simulink model "Environment"  (R2012b)
settings: Solver=FixedStepDiscrete  StartTime=0.0  StopTime=500  FixedStep=0.1  RelTol=1e-3
values from neighbouring files (symbols this model uses):
  tank1_cross_section_area_m2 = 1    [constants.m]
  tank1_max_vol_m3 = 7    [constants.m]
  tank1_pump_flow_rate_m3s = 0.2    [constants.m]
  tank1_sensor_hi_height_m = 5    [constants.m]
  tank1_sensor_lo_height_m = 2    [constants.m]
  tank1_valve_flow_rate_m3s = 0.1    [constants.m]
  tank2_cross_section_area_m2 = 2    [constants.m]
  tank2_e_valve_flow_rate_m3s = 0.2    [constants.m]
  tank2_max_vol_m3 = 8    [constants.m]
  tank2_p_valve_flow_rate_m3s = 0.05    [constants.m]
  tank2_sensor_hi_height_m = 3    [constants.m]
  tank2_sensor_lo_height_m = 1    [constants.m]
  tank2_sensor_md_height_m = 2    [constants.m]
  time_increment_s = 0.1    [constants.m]
settings Model: Creator=Kerianne  LastModifiedBy=Kerianne
settings DataIOCC: SaveFormat=Structure
settings OptimizationCC: InlineParams=on

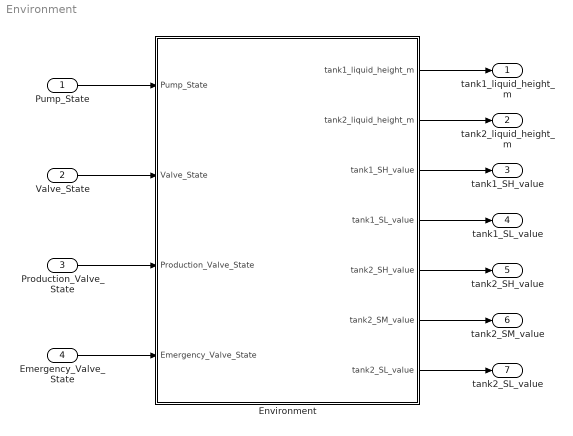
== system Environment ==
  Pump_State : Inport
  Valve_State : Inport  Port=2
  Production_Valve_State : Inport  Port=3
  Emergency_Valve_State : Inport  Port=4
  Environment : Subsystem
  tank1_liquid_height_m : Outport
  tank2_liquid_height_m : Outport  Port=2
  tank1_SH_value : Outport  Port=3
  tank1_SL_value : Outport  Port=4
  tank2_SH_value : Outport  Port=5
  tank2_SM_value : Outport  Port=6
  tank2_SL_value : Outport  Port=7
  wires:
  Pump_State/1 -> Environment/1(Pump_State)
  Valve_State/1 -> Environment/2(Valve_State)
  Production_Valve_State/1 -> Environment/3(Production_Valve_State)
  Emergency_Valve_State/1 -> Environment/4(Emergency_Valve_State)
  Environment/1(tank1_liquid_height_m) -> tank1_liquid_height_m/1
  Environment/2(tank2_liquid_height_m) -> tank2_liquid_height_m/1
  Environment/3(tank1_SH_value) -> tank1_SH_value/1
  Environment/4(tank1_SL_value) -> tank1_SL_value/1
  Environment/5(tank2_SH_value) -> tank2_SH_value/1
  Environment/6(tank2_SM_value) -> tank2_SM_value/1
  Environment/7(tank2_SL_value) -> tank2_SL_value/1

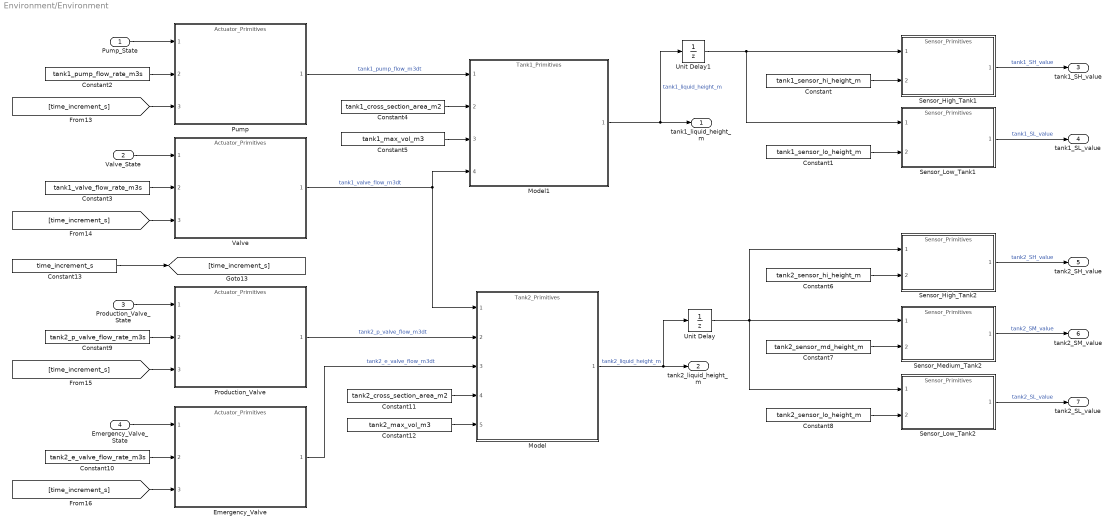
== system Environment/Environment ==
  Pump_State : Inport
  Valve_State : Inport  Port=2
  Production_Valve_State : Inport  Port=3
  Emergency_Valve_State : Inport  Port=4
  Constant : Constant  Value=tank1_sensor_hi_height_m
  Constant1 : Constant  Value=tank1_sensor_lo_height_m
  Constant10 : Constant  Value=tank2_e_valve_flow_rate_m3s
  Constant11 : Constant  Value=tank2_cross_section_area_m2
  Constant12 : Constant  Value=tank2_max_vol_m3
  Constant13 : Constant  Value=time_increment_s
  Constant2 : Constant  Value=tank1_pump_flow_rate_m3s
  Constant3 : Constant  Value=tank1_valve_flow_rate_m3s
  Constant4 : Constant  Value=tank1_cross_section_area_m2
  Constant5 : Constant  Value=tank1_max_vol_m3
  Constant6 : Constant  Value=tank2_sensor_hi_height_m
  Constant7 : Constant  Value=tank2_sensor_md_height_m
  Constant8 : Constant  Value=tank2_sensor_lo_height_m
  Constant9 : Constant  Value=tank2_p_valve_flow_rate_m3s
  Emergency_Valve : ModelReference  ModelNameDialog=Actuator_Primitives  SimulationMode=Normal  ModelReferenceVersion=1.26  CopyOfModelName=Actuator_Primitives  DefaultDataLogging=on
  Model : ModelReference  ModelNameDialog=Tank2_Primitives  SimulationMode=Normal  ModelReferenceVersion=1.32  CopyOfModelName=Tank2_Primitives  DefaultDataLogging=on
  Model1 : ModelReference  ModelNameDialog=Tank1_Primitives  SimulationMode=Normal  ModelReferenceVersion=1.30  CopyOfModelName=Tank1_Primitives  DefaultDataLogging=on
  Production_Valve : ModelReference  ModelNameDialog=Actuator_Primitives  SimulationMode=Normal  ModelReferenceVersion=1.26  CopyOfModelName=Actuator_Primitives  DefaultDataLogging=on
  Pump : ModelReference  ModelNameDialog=Actuator_Primitives  SimulationMode=Normal  ModelReferenceVersion=1.26  CopyOfModelName=Actuator_Primitives  DefaultDataLogging=on
  Sensor_High_Tank1 : ModelReference  ModelNameDialog=Sensor_Primitives  SimulationMode=Normal  ModelReferenceVersion=1.33  CopyOfModelName=Sensor_Primitives  DefaultDataLogging=on
  Sensor_High_Tank2 : ModelReference  ModelNameDialog=Sensor_Primitives  SimulationMode=Normal  ModelReferenceVersion=1.33  CopyOfModelName=Sensor_Primitives  DefaultDataLogging=on
  Sensor_Low_Tank1 : ModelReference  ModelNameDialog=Sensor_Primitives  SimulationMode=Normal  ModelReferenceVersion=1.33  CopyOfModelName=Sensor_Primitives  DefaultDataLogging=on
  Sensor_Low_Tank2 : ModelReference  ModelNameDialog=Sensor_Primitives  SimulationMode=Normal  ModelReferenceVersion=1.33  CopyOfModelName=Sensor_Primitives  DefaultDataLogging=on
  Sensor_Medium_Tank2 : ModelReference  ModelNameDialog=Sensor_Primitives  SimulationMode=Normal  ModelReferenceVersion=1.33  CopyOfModelName=Sensor_Primitives  DefaultDataLogging=on
  Unit Delay : UnitDelay  SampleTime=-1
  Unit Delay1 : UnitDelay  SampleTime=-1
  Valve : ModelReference  ModelNameDialog=Actuator_Primitives  SimulationMode=Normal  ModelReferenceVersion=1.26  CopyOfModelName=Actuator_Primitives  DefaultDataLogging=on
  tank1_liquid_height_m : Outport
  tank2_liquid_height_m : Outport  Port=2
  tank1_SH_value : Outport  Port=3
  tank1_SL_value : Outport  Port=4
  tank2_SH_value : Outport  Port=5
  tank2_SM_value : Outport  Port=6
  tank2_SL_value : Outport  Port=7
  wires:
  Sensor_Low_Tank2/1 -> tank2_SL_value/1  "tank2_SL_value"
  Sensor_Medium_Tank2/1 -> tank2_SM_value/1  "tank2_SM_value"
  Sensor_Low_Tank1/1 -> tank1_SL_value/1  "tank1_SL_value"
  Sensor_High_Tank2/1 -> tank2_SH_value/1  "tank2_SH_value"
  Sensor_High_Tank1/1 -> tank1_SH_value/1  "tank1_SH_value"
  Constant2/1 -> Pump/2
  Constant3/1 -> Valve/2
  Unit Delay/1 -> Sensor_High_Tank2/1, Sensor_Medium_Tank2/1, Sensor_Low_Tank2/1
  Constant1/1 -> Sensor_Low_Tank1/2
  Constant/1 -> Sensor_High_Tank1/2
  Constant11/1 -> Model/4
  Constant4/1 -> Model1/2
  [time_increment_s] -> Valve/3
  [time_increment_s] -> Emergency_Valve/3
  [time_increment_s] -> Pump/3
  [time_increment_s] -> Production_Valve/3
  Constant9/1 -> Production_Valve/2
  Valve/1 -> Model1/4, Model/1  "tank1_valve_flow_m3dt"
  Production_Valve/1 -> Model/2  "tank2_p_valve_flow_m3dt"
  Constant10/1 -> Emergency_Valve/2
  Valve_State/1 -> Valve/1
  Emergency_Valve_State/1 -> Emergency_Valve/1
  Pump_State/1 -> Pump/1
  Production_Valve_State/1 -> Production_Valve/1
  Pump/1 -> Model1/1  "tank1_pump_flow_m3dt"
  Constant12/1 -> Model/5
  Constant5/1 -> Model1/3
  Model1/1 -> Unit Delay1/1, tank1_liquid_height_m/1  "tank1_liquid_height_m"
  Model/1 -> tank2_liquid_height_m/1, Unit Delay/1  "tank2_liquid_height_m"
  Constant8/1 -> Sensor_Low_Tank2/2
  Constant13/1 -> [time_increment_s]
  Constant6/1 -> Sensor_High_Tank2/2
  Constant7/1 -> Sensor_Medium_Tank2/2
  Emergency_Valve/1 -> Model/3  "tank2_e_valve_flow_m3dt"
  Unit Delay1/1 -> Sensor_Low_Tank1/1, Sensor_High_Tank1/1
